simulink model "case123_30dsimulink"  (R2013a)
settings: Solver=ode3  SolverMode=SingleTasking  StartTime=7.22  StopTime=95.04  FixedStep=.02  RelTol=1e-3
values from neighbouring files (symbols this model uses):
  b = 0.001:.002:.02    [Num4s.m]    (also in cont.m = 0.001:0.002:0.04; lab2case1.m = 2*zeta*wn*.1389*x^2; lab2case1change.m = 2*zeta*wn*.1389*x^2; num2.m = 0.002:0.0008:0.04)
undefined symbols (not defined in the file or in its folder): init
settings Model: Creator=guilh_000  LastModifiedBy=z
settings DataIOCC: SignalLoggingSaveFormat=ModelDataLogs
settings OptimizationCC: BlockReduction=off  BooleanDataType=off
settings DebuggingCC: SaveWithParameterizedLinksMsg=none  SignalResolutionControl=TryResolveAllWithWarning  SolverPrmCheckMsg=none  MultiTaskDSMMsg=warning  MultiTaskCondExecSysMsg=none  StrictBusMsg=None
settings HardwareCC: TargetUnknown=on
settings RTWCC: IncludeERTFirstTime=on

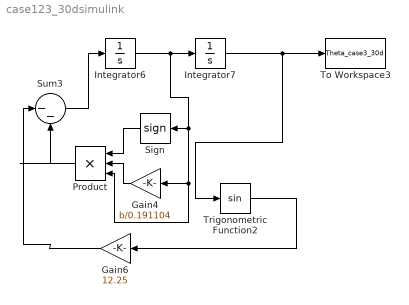
== system case123_30dsimulink ==
  Gain4 : Gain  Gain=b/0.191104
  Gain6 : Gain  Gain=12.25
  Integrator6 : Integrator
  Integrator7 : Integrator  InitialCondition=init
  Product : Product  Inputs=3
  Sign : Signum
  Sum3 : Sum  Inputs=|--
  To Workspace3 : ToWorkspace  VariableName=Theta_case3_30d  SampleTime=-1
  Trigonometric Function2 : Trigonometry
  wires:
  Sum3/1 -> Integrator6/1
  Gain6/1 -> Sum3/1
  Integrator7/1 -> Trigonometric Function2/1, To Workspace3/1
  Trigonometric Function2/1 -> Gain6/1
  Product/1 -> Sum3/2
  Sign/1 -> Product/1
  Gain4/1 -> Product/2
  Integrator6/1 -> Product/3, Gain4/1, Sign/1, Integrator7/1
